simulink model "dcMotorSim"  (R2023b)
settings: Solver=VariableStepAuto  StartTime=0.0  StopTime=10  RelTol=1e-3
values from neighbouring files (symbols this model uses):
  J = 0.181    [dcMotorPar.m]
  kb = 36.9e-3    (= 0.0369)    [dcMotorPar.m]
  kf = 0.1    [dcMotorPar.m]
  km = 20    [dcMotorPar.m]
  L = 0.463e-3    (= 0.000463)    [dcMotorPar.m]
  R = 0.608    [dcMotorPar.m]
settings Model: Creator=chsl  LastModifiedBy=jacob
settings SolverCC: AlgebraicLoopSolver=TrustRegion
settings DataIOCC: ReturnWorkspaceOutputs=off
settings DebuggingCC: UnconnectedInputMsg=warning  UnconnectedOutputMsg=warning  UnconnectedLineMsg=warning  ArithmeticOperatorsInVariantConditions=warning
settings ModelReferenceCC: EnableRefExpFcnMdlSchedulingChecks=on
settings SFSimCC: SimUseLocalCustomCode=off  CustomCodeUndefinedFunction=UseInterfaceOnly
settings RTWCC: RTWUseLocalCustomCode=off

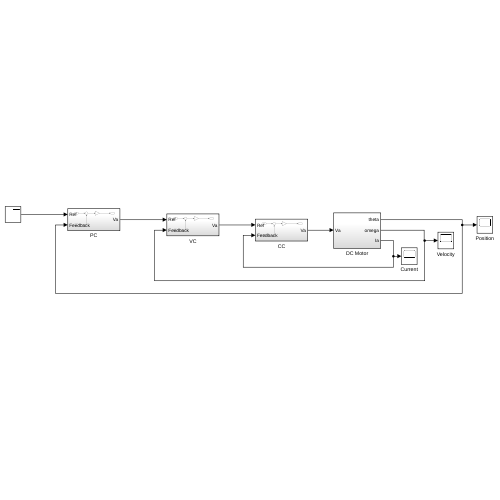
[thumbnail: Simulink's stored preview of the top-level diagram]
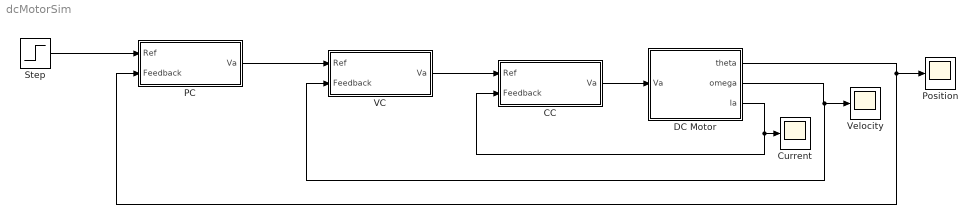
== system dcMotorSim ==
  CC : Subsystem
  Current : Scope
  DC Motor : Subsystem
  PC : Subsystem
  Position : Scope
  Step : Step  SampleTime=0
  VC : Subsystem
  Velocity : Scope
  wires:
  DC Motor/3(Ia) -> CC/2(Feedback), Current/1
  CC/1(Va) -> DC Motor/1(Va)
  VC/1(Va) -> CC/1(Ref)
  PC/1(Va) -> VC/1(Ref)
  Step/1 -> PC/1(Ref)
  DC Motor/1(theta) -> Position/1, PC/2(Feedback)
  DC Motor/2(omega) -> VC/2(Feedback), Velocity/1

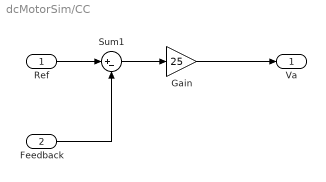
== system dcMotorSim/CC ==
  Ref : Inport
  Feedback : Inport  Port=2
  Gain : Gain  Gain=25
  Sum1 : Sum  Inputs=|+-
  Va : Outport
  wires:
  Feedback/1 -> Sum1/2
  Ref/1 -> Sum1/1
  Sum1/1 -> Gain/1
  Gain/1 -> Va/1

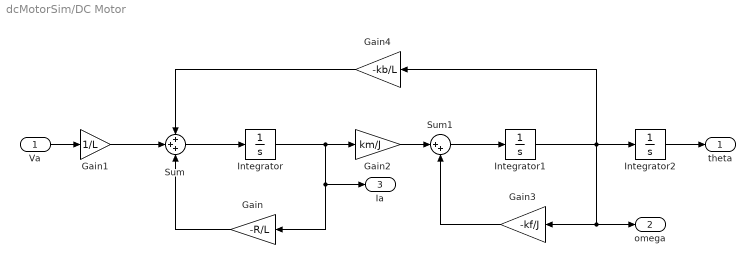
== system dcMotorSim/DC Motor ==
  Va : Inport
  Gain : Gain  Gain=-R/L
  Gain1 : Gain  Gain=1/L
  Gain2 : Gain  Gain=km/J
  Gain3 : Gain  Gain=-kf/J
  Gain4 : Gain  Gain=-kb/L
  Integrator : Integrator
  Integrator1 : Integrator
  Integrator2 : Integrator
  Sum : Sum  Inputs=+++
  Sum1 : Sum  Inputs=|++
  theta : Outport  VectorParamsAs1DForOutWhenUnconnected=off
  omega : Outport  Port=2  VectorParamsAs1DForOutWhenUnconnected=off
  Ia : Outport  Port=3  VectorParamsAs1DForOutWhenUnconnected=off
  wires:
  Gain2/1 -> Sum1/1
  Integrator1/1 -> Gain4/1, omega/1, Gain3/1, Integrator2/1
  Integrator/1 -> Ia/1, Gain/1, Gain2/1
  Sum/1 -> Integrator/1
  Va/1 -> Gain1/1
  Gain1/1 -> Sum/2
  Gain3/1 -> Sum1/2
  Integrator2/1 -> theta/1
  Gain4/1 -> Sum/1
  Sum1/1 -> Integrator1/1
  Gain/1 -> Sum/3

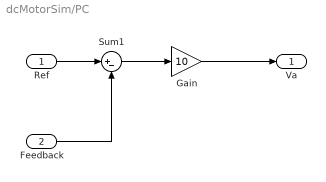
== system dcMotorSim/PC ==
  Ref : Inport
  Feedback : Inport  Port=2
  Gain : Gain  Gain=10
  Sum1 : Sum  Inputs=|+-
  Va : Outport
  wires:
  Feedback/1 -> Sum1/2
  Ref/1 -> Sum1/1
  Sum1/1 -> Gain/1
  Gain/1 -> Va/1

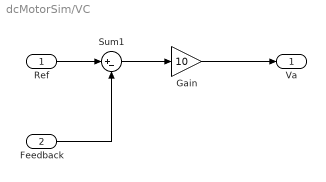
== system dcMotorSim/VC ==
  Ref : Inport
  Feedback : Inport  Port=2
  Gain : Gain  Gain=10
  Sum1 : Sum  Inputs=|+-
  Va : Outport
  wires:
  Feedback/1 -> Sum1/2
  Ref/1 -> Sum1/1
  Sum1/1 -> Gain/1
  Gain/1 -> Va/1
